simulink model "Simple"  (R2024b)
settings: Solver=VariableStepAuto  StartTime=0.0  StopTime=25.3849  MaxStep=.001  RelTol=1e-3
libraries: simulink x1
settings Model: Creator=hjhje  LastModifiedBy=hjhje

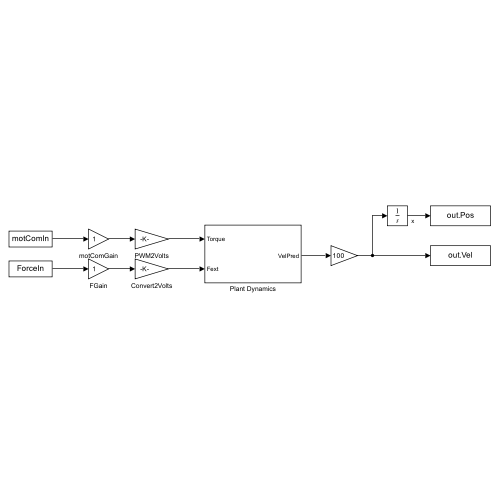
[thumbnail: Simulink's stored preview of the top-level diagram]
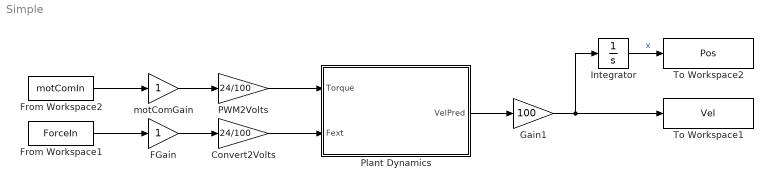
== system Simple ==
  Convert2Volts : Gain  Gain=24/100
  FGain : Gain
  From Workspace1 : FromWorkspace  VariableName=ForceIn  SampleTime=-1  Interpolate=off  OutputAfterFinalValue=Holding final value
  From Workspace2 : FromWorkspace  VariableName=motComIn  SampleTime=-1  Interpolate=off  OutputAfterFinalValue=Holding final value
  Gain1 : Gain  Gain=100
  Integrator : Integrator
  PWM2Volts : Gain  Gain=24/100
  Plant Dynamics : Subsystem
  To Workspace1 : ToWorkspace  VariableName=Vel  SaveFormat=Timeseries  SampleTime=-1
  To Workspace2 : ToWorkspace  VariableName=Pos  SaveFormat=Timeseries  SampleTime=-1
  motComGain : Gain
  wires:
  From Workspace2/1 -> motComGain/1
  From Workspace1/1 -> FGain/1
  Plant Dynamics/1(VelPred) -> Gain1/1
  Gain1/1 -> Integrator/1, To Workspace1/1
  Integrator/1 -> To Workspace2/1  "x"
  motComGain/1 -> PWM2Volts/1
  FGain/1 -> Convert2Volts/1
  PWM2Volts/1 -> Plant Dynamics/1(Torque)
  Convert2Volts/1 -> Plant Dynamics/2(Fext)

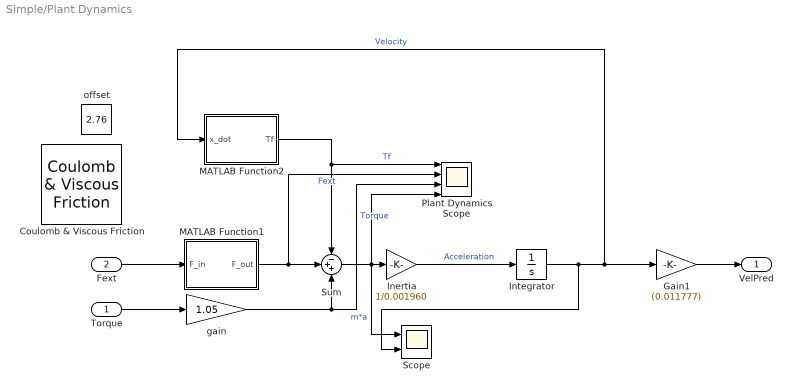
== system Simple/Plant Dynamics ==
  Torque : Inport
  Fext : Inport  Port=2
  Coulomb & Viscous Friction : simulink/Discontinuities/Coulomb & Viscous Friction  offset=10.95*24/100  gain=1/0.090977
  Gain1 : Gain  Gain=(0.011777)
  Inertia : Gain  Gain=1/0.001960
  Integrator : Integrator
  MATLAB Function1 : MATLAB Function  TreatAsAtomicUnit=on
  MATLAB Function2 : MATLAB Function  TreatAsAtomicUnit=on
  Plant Dynamics Scope : Scope  NumInputPorts=4
  Scope : Scope  NumInputPorts=2
  Sum : Sum  Inputs=-++
  gain : Gain  Gain=1.05
  offset : Constant  Value=2.76
  VelPred : Outport
  wires:
  Inertia/1 -> Integrator/1  "Acceleration"
  Sum/1 -> Scope/1, Plant Dynamics Scope/4, Inertia/1  "m*a"
  MATLAB Function2/1(Tf) -> Sum/1, Plant Dynamics Scope/1  "Tf"
  Integrator/1 -> Scope/2, MATLAB Function2/1(x_dot), Gain1/1  "Velocity"
  Torque/1 -> gain/1
  Fext/1 -> MATLAB Function1/1(F_in)
  MATLAB Function1/1(F_out) -> Plant Dynamics Scope/2, Sum/2  "Fext"
  gain/1 -> Plant Dynamics Scope/3, Sum/3  "Torque"
  Gain1/1 -> VelPred/1

== matlab function Simple/Plant Dynamics/MATLAB Function2 ==
  data: x_dot input; Tf output
function Tf = fcn(x_dot)

%old viscousGain = .8*(1.0 / 0.090977); % 10.992
% viscousGain = 1.5*(1.0 / 0.090977);
% viscousGain = 9.873644121;
% viscousGain = (1/0.098736441);
viscousGain = 1.65*0.1163;

coulombGain = 1;
if (x_dot > 0)
    coulombGain = 10.95;
else
    coulombGain = .95*10.95;
end
Tf = 1*viscousGain*x_dot + 1*coulombGain*(24/100)*tanh(150*x_dot);

== matlab function Simple/Plant Dynamics/MATLAB Function1 ==
  data: F_in input; F_out output
function F_out = fcn(F_in)

if (F_in > 0)
    scale = 1.0;
else
    scale = 1;
end
% scale =.8;
F_out = scale*F_in;
